simulink model "PID_Circular"  (R2018b)
settings: Solver=VariableStepAuto  StartTime=0.0  StopTime=10.0  RelTol=1e-3
values from neighbouring files (symbols this model uses):
  x0 = 1    [init_handle.m]
  y0 = 1    [init_handle.m]
libraries: simulink x1
settings Model: Creator=giga4  LastModifiedBy=giga4

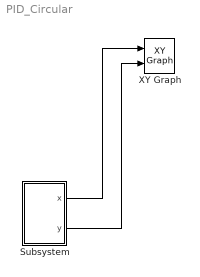
== system PID_Circular ==
  Subsystem : Subsystem
  XY Graph : simulink/Sinks/XY Graph  xmin=x_L  xmax=x_R  ymin=y_D  ymax=y_U  st=-1
  wires:
  Subsystem/2(y) -> XY Graph/2
  Subsystem/1(x) -> XY Graph/1

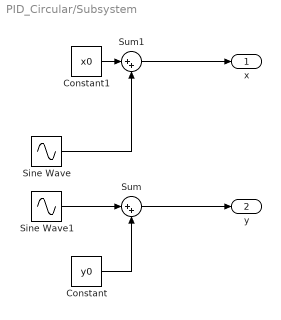
== system PID_Circular/Subsystem ==
  Constant : Constant  Value=y0
  Constant1 : Constant  Value=x0
  Sine Wave : Sin  SampleTime=0
  Sine Wave1 : Sin  Phase=pi/2  SampleTime=0
  Sum : Sum  Inputs=|++
  Sum1 : Sum  Inputs=|++
  x : Outport
  y : Outport  Port=2
  wires:
  Sum/1 -> y/1
  Sine Wave1/1 -> Sum/1
  Sine Wave/1 -> Sum1/2
  Constant1/1 -> Sum1/1
  Constant/1 -> Sum/2
  Sum1/1 -> x/1
